simulink model "suspension_experiment"  (R2026a)
settings: Solver=VariableStepAuto  StopTime=1000.0
undefined symbols (not defined in the file): filter_param, r_param
libraries: lib_sensors x3, lib_plant x1
settings Model: Creator=alessandro-nardin  LastModifiedBy=fiore

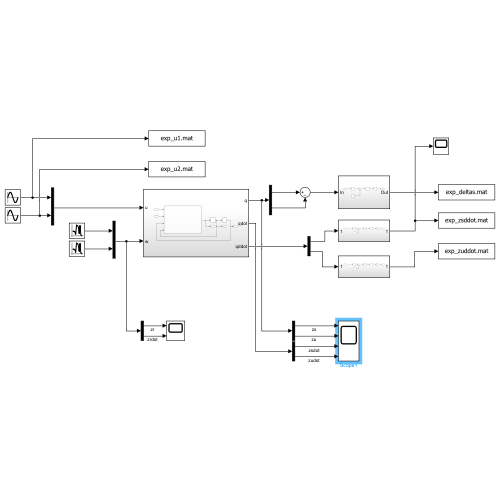
[thumbnail: Simulink's stored preview of the top-level diagram]
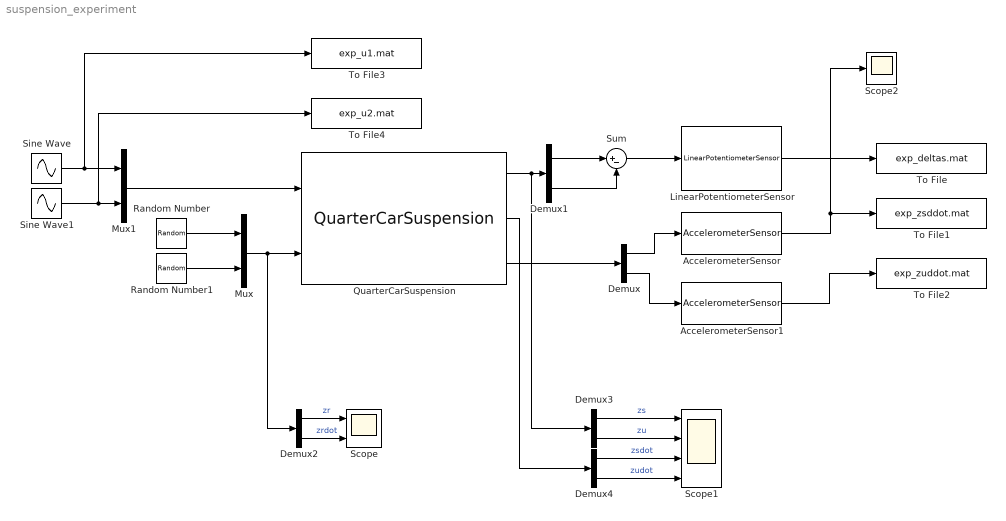
== system suspension_experiment ==
  AccelerometerSensor : lib_sensors/AccelerometerSensor  SystemSampleTime=-1  VariantActivationTime=update diagram  EmptyChoice=off  PassThrough=off  PassThroughVariantControl=(default)  EmptyChoiceVariantControl=(default)  AllowFlexibleInterface=on  Latency=0  AutoFrameSizeCalculation=off
  AccelerometerSensor1 : lib_sensors/AccelerometerSensor  SystemSampleTime=-1  VariantActivationTime=update diagram  EmptyChoice=off  PassThrough=off  PassThroughVariantControl=(default)  EmptyChoiceVariantControl=(default)  AllowFlexibleInterface=on  Latency=0  AutoFrameSizeCalculation=off
  Demux{,1..4} (5 alike) : Demux  Outputs=2
  LinearPotentiometerSensor : lib_sensors/LinearPotentiometerSensor  SystemSampleTime=-1  VariantActivationTime=update diagram  EmptyChoice=off  PassThrough=off  PassThroughVariantControl=(default)  EmptyChoiceVariantControl=(default)  AllowFlexibleInterface=on  Latency=0  AutoFrameSizeCalculation=off
  Mux : Mux  Inputs=2
  Mux1 : Mux  Inputs=2
  QuarterCarSuspension : lib_plant/QuarterCarSuspension  SystemSampleTime=-1  VariantActivationTime=update diagram  EmptyChoice=off  PassThrough=off  PassThroughVariantControl=(default)  EmptyChoiceVariantControl=(default)  AllowFlexibleInterface=on  Latency=0  AutoFrameSizeCalculation=off
      settings: SourceProductName=Lib Plant
  Random Number : RandomNumber  Variance=r_param.rz_var  SampleTime=0
  Random Number1 : RandomNumber  Variance=r_param.rzdot_var  Seed=1  SampleTime=0
  Scope : Scope  NumInputPorts=2
      settings: ActiveDisplayYMinimum=-0.96948852617779024  ActiveDisplayYMaximum=0.9567756425914673
  Scope1 : Scope  NumInputPorts=4
      settings: ActiveDisplayYMinimum=-0.082678659114851935  ActiveDisplayYMaximum=0.08056249888067496
  Scope2 : Scope
      settings: ActiveDisplayYMinimum=-2.8526927947998049  ActiveDisplayYMaximum=2.6221721649169925  DataLoggingVariableName=ScopeData2
  Sine Wave : Sin  Amplitude=0  Frequency=0.5  SampleTime=0
  Sine Wave1 : Sin  Amplitude=0  SampleTime=0
  Sum : Sum  Inputs=|+-
  To File : ToFile  Filename=exp_deltas.mat  MatrixName=deltas  SampleTime=filter_param.sample_t
  To File1 : ToFile  Filename=exp_zsddot.mat  MatrixName=zsddot  SampleTime=filter_param.sample_t
  To File2 : ToFile  Filename=exp_zuddot.mat  MatrixName=zuddot  SampleTime=filter_param.sample_t
  To File3 : ToFile  Filename=exp_u1.mat  MatrixName=u1  SampleTime=filter_param.sample_t
  To File4 : ToFile  Filename=exp_u2.mat  MatrixName=u2  SampleTime=filter_param.sample_t
  wires:
  Demux/1 -> AccelerometerSensor/1
  Demux/2 -> AccelerometerSensor1/1
  QuarterCarSuspension/3 -> Demux/1
  Demux1/1 -> Sum/1
  Demux1/2 -> Sum/2
  Sum/1 -> LinearPotentiometerSensor/1
  LinearPotentiometerSensor/1 -> To File/1
  AccelerometerSensor/1 -> Scope2/1, To File1/1
  AccelerometerSensor1/1 -> To File2/1
  Random Number/1 -> Mux/1
  Random Number1/1 -> Mux/2
  Mux1/1 -> QuarterCarSuspension/1
  Demux2/2 -> Scope/2  "zrdot"
  Demux2/1 -> Scope/1  "zr"
  QuarterCarSuspension/2 -> Demux4/1
  Demux3/1 -> Scope1/1  "zs"
  Demux4/2 -> Scope1/4  "zudot"
  Demux3/2 -> Scope1/2  "zu"
  Demux4/1 -> Scope1/3  "zsdot"
  QuarterCarSuspension/1 -> Demux3/1, Demux1/1
  Mux/1 -> Demux2/1, QuarterCarSuspension/2
  Sine Wave1/1 -> To File4/1, Mux1/2
  Sine Wave/1 -> To File3/1, Mux1/1
